simulink model "Insulin_Subsystem"  (R2018a)
settings: Solver=VariableStepAuto  StartTime=0.0  StopTime=10.0  RelTol=1e-3
settings Model: Creator=cgonterman  LastModifiedBy=cgonterman

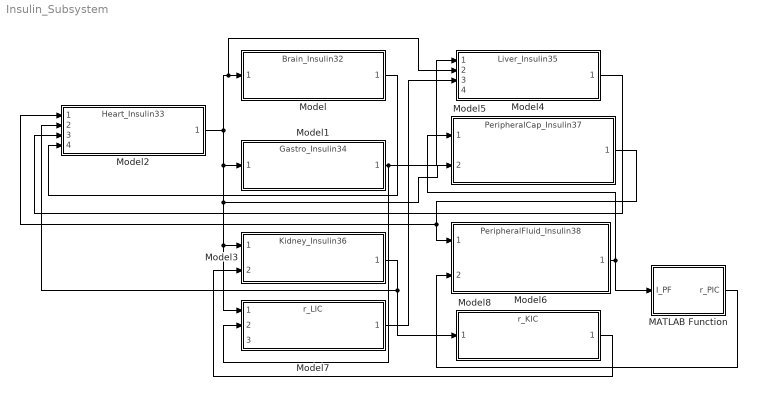
== system Insulin_Subsystem ==
  MATLAB Function : MATLAB Function  TreatAsAtomicUnit=on
  Model : ModelReference  ModelNameDialog=Brain_Insulin32  SimulationMode=Normal  ModelReferenceVersion=1.2
  Model1 : ModelReference  ModelNameDialog=Gastro_Insulin34  SimulationMode=Normal  ModelReferenceVersion=1.2
  Model2 : ModelReference  ModelNameDialog=Heart_Insulin33  SimulationMode=Normal  ModelReferenceVersion=1.3
  Model3 : ModelReference  ModelNameDialog=Kidney_Insulin36  SimulationMode=Normal  ModelReferenceVersion=1.3
  Model4 : ModelReference  ModelNameDialog=Liver_Insulin35  SimulationMode=Normal  ModelReferenceVersion=1.3
  Model5 : ModelReference  ModelNameDialog=PeripheralCap_Insulin37  SimulationMode=Normal  ModelReferenceVersion=1.3
  Model6 : ModelReference  ModelNameDialog=PeripheralFluid_Insulin38  SimulationMode=Normal  ModelReferenceVersion=1.3
  Model7 : ModelReference  ModelNameDialog=r_LIC  SimulationMode=Normal  ModelReferenceVersion=1.2
  Model8 : ModelReference  ModelNameDialog=r_KIC  SimulationMode=Normal  ModelReferenceVersion=1.1
  wires:
  Model2/1 -> Model7/1, Model3/1, Model5/2, Model1/1, Model4/2, Model/1
  Model/1 -> Model2/4
  Model4/1 -> Model2/3
  Model3/1 -> Model8/1, Model2/2
  Model1/1 -> Model7/2, Model4/1
  Model5/1 -> Model2/1, Model6/1
  Model6/1 -> MATLAB Function/1(I_PF), Model5/1
  Model7/1 -> Model4/3
  Model8/1 -> Model3/2
  MATLAB Function/1(r_PIC) -> Model6/2

== matlab function Insulin_Subsystem/MATLAB Function ==
  data: I_PF input; r_PIC output
function r_PIC = fcn(I_PF)
r_PIC=I_PF/(((1-0.15)/(0.15*Q_i_P))-(20/V_i_PF));
